simulink subsystem "quarter_suspension_subsystem"  (R2020b)
settings: Solver=VariableStepAuto  StartTime=0.0  StopTime=10.0  RelTol=1e-3
settings Model: Creator=Ricky  LastModifiedBy=Ricky

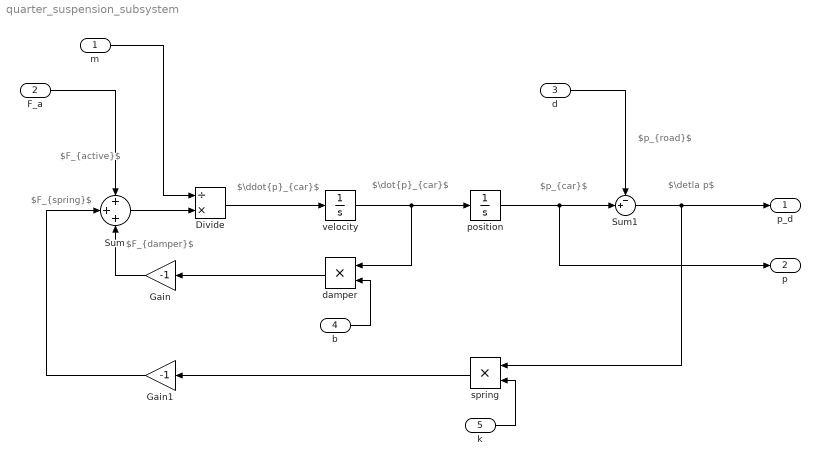
== system quarter_suspension_subsystem ==
  note: $F_{spring}$
  note: $F_{damper}$
  note: $F_{active}$
  note: $p_{road}$
  note: $p_{car}$
  note: $\detla p$
  note: $\dot{p}_{car}$
  note: $\ddot{p}_{car}$
  m : Inport  Tag=m
  F_a : Inport  Tag=F_a  Port=2
  d : Inport  Tag=d  Port=3
  b : Inport  Tag=b  Port=4
  k : Inport  Tag=k  Port=5
  Divide : Product  Inputs=/*
  Gain : Gain  Gain=-1
  Gain1 : Gain  Gain=-1
  Sum : Sum  Inputs=+++
  Sum1 : Sum  Inputs=-+|
  damper : Product
  position : Integrator
  spring : Product
  velocity : Integrator
  p_d : Outport  Tag=p_d
  p : Outport  Tag=p  Port=2
  wires:
  Gain1/1 -> Sum/2
  Divide/1 -> velocity/1
  position/1 -> Sum1/2, p/1
  spring/1 -> Gain1/1
  Sum1/1 -> spring/1, p_d/1
  b/1 -> damper/2
  damper/1 -> Gain/1
  velocity/1 -> position/1, damper/1
  Sum/1 -> Divide/2
  Gain/1 -> Sum/3
  d/1 -> Sum1/1
  F_a/1 -> Sum/1
  k/1 -> spring/2
  m/1 -> Divide/1
